simulink model "my_gm_HDLPayloadFull"  (R2024a)
settings: Solver=FixedStepDiscrete  StartTime=0.0  StopTime=stopTime  RelTol=1e-3
values from neighbouring files (symbols this model uses):
  pWords = [pWords binl2str(pBitsRaw{i})]    [testPayloadFull.m]
undefined symbols (not defined in the file or in its folder): fs, msgIn
libraries: hdlmdlgenlib x66, hdlsllib x16, dspsrcs4 x9, dspsigops x9, simulink x4, whdlutilities x4, whdledac x1
(part 1 of 2)
settings Model: SimulationMode=accelerator  Creator=cotti  LastModifiedBy=cotti
settings OptimizationCC: BlockReduction=off  ConditionallyExecuteInputs=off  DefaultParameterBehavior=Inlined  InheritOutputTypeSmallerThanSingle=on
settings DebuggingCC: AlgebraicLoopMsg=error  ArtificialAlgebraicLoopMsg=error  InheritedTsInSrcMsg=none  SingleTaskRateTransMsg=error  UnconnectedInputMsg=warning  UnconnectedOutputMsg=warning  UnconnectedLineMsg=warning
settings HardwareCC: ProdBitPerPointer=32  ProdBitPerSizeT=32  ProdBitPerPtrDiffT=32  ProdLargestAtomicFloat=None  ProdIntDivRoundTo=Undefined  ProdEndianess=Unspecified  ProdWordSize=32  ProdHWDeviceType=ASIC/FPGA->ASIC/FPGA  TargetBitPerLong=64  TargetBitPerPointer=64  TargetBitPerSizeT=64  TargetBitPerPtrDiffT=64  TargetLongLongMode=on  TargetIntDivRoundTo=Zero  TargetEndianess=LittleEndian  TargetWordSize=64  TargetHWDeviceType=Custom Processor->MATLAB Host Computer  ProdEqTarget=off

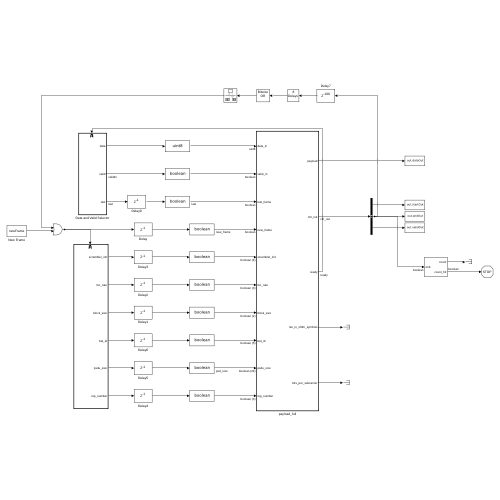
[thumbnail: Simulink's stored preview of the top-level diagram]
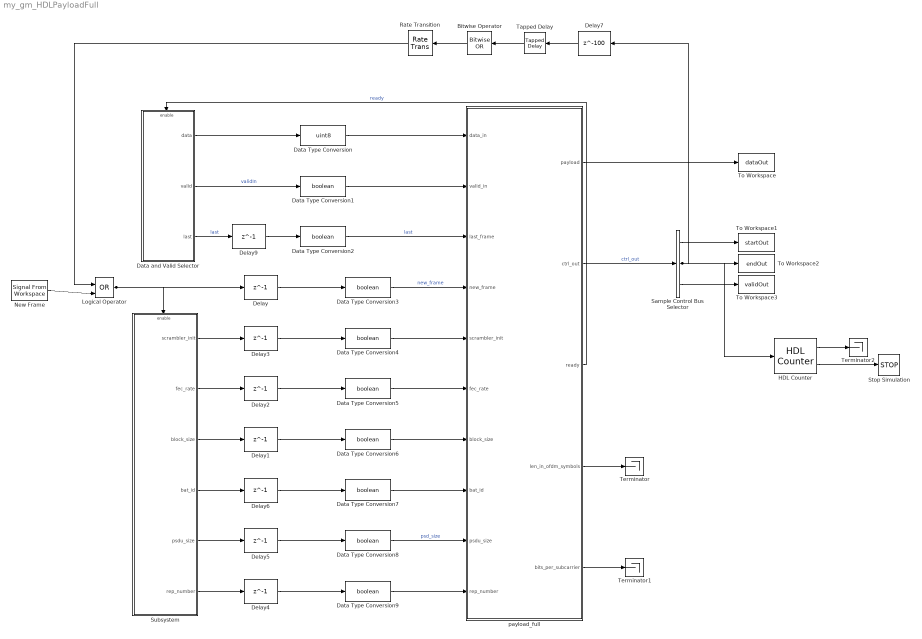
== system my_gm_HDLPayloadFull ==
  Bitwise Operator : simulink/Logic and Bit Operations/Bitwise Operator  logicop=OR  UseBitMask=off  BitMask=bin2dec('11011001')  BitMaskRealWorld=Stored Integer
      settings: LibrarySourceBlock=|
      | hdlsllib/Logic and Bit
      | Operations/Bitwise
      | Operator
  Data Type Conversion : DataTypeConversion  OutDataTypeStr=uint8  SaturateOnIntegerOverflow=off  RndMeth=Floor
  Data Type Conversion{1..9} (9 alike) : DataTypeConversion  OutDataTypeStr=boolean  SaturateOnIntegerOverflow=off  RndMeth=Floor
  Data and Valid Selector : Subsystem  TreatAsAtomicUnit=on
  Delay{,1..6,9} (8 alike) : Delay  DelayLength=1  InitialCondition=0  UseCircularBuffer=on
  Delay7 : Delay  DelayLength=100  InitialCondition=0  UseCircularBuffer=on
  HDL Counter : hdlsllib/Sources/HDL Counter  CountType=Count limited  CountInit=0  CountStep=1  CountMax=length(msgIn)  CountFromType=Initial value  CountFrom=0  CountResetPort=off  CountLoadPort=off  CountEnbPort=on  CountDirPort=off  CountHitOutputPort=on  CountDataType=Unsigned  CountWordLen=8  CountFracLen=0  CountSampTime=1
  Logical Operator : Logic  Operator=OR  IconShape=distinctive  AllPortsSameDT=off  OutDataTypeStr=boolean
  New Frame : dspsrcs4/Signal From Workspace  X=newFrame  Ts=8/fs  nsamps=1  OutputAfterFinalValue=Setting to zero  ignoreOrWarnInputAndFrameLengths=off  OutputFrames=off
  Rate Transition : RateTransition  OutPortSampleTimeOpt=Multiple of input port sample time  OutPortSampleTimeMultiple=8
  Sample Control Bus Selector : whdlutilities/Sample Control Bus Selector  OutputSignals=start,end,valid
  Stop Simulation : Stop
  Subsystem : Subsystem
  Tapped Delay : simulink/Discrete/Tapped Delay  vinit=0.0  samptime=-1  NumDelays=8  DelayOrder=Oldest  includeCurrent=off
      settings: LibrarySourceBlock=hdlsllib/Discrete/Tapped Delay
  Terminator : Terminator
  Terminator1 : Terminator
  Terminator2 : Terminator
  To Workspace : ToWorkspace  VariableName=dataOut  SampleTime=1/fs
      settings: Save2DSignal=2-D array (concatenate along first dimension)
  To Workspace1 : ToWorkspace  VariableName=startOut  SampleTime=1/fs
      settings: Save2DSignal=2-D array (concatenate along first dimension)
  To Workspace2 : ToWorkspace  VariableName=endOut  SampleTime=1/fs
      settings: Save2DSignal=2-D array (concatenate along first dimension)
  To Workspace3 : ToWorkspace  VariableName=validOut  SampleTime=1/fs
      settings: Save2DSignal=2-D array (concatenate along first dimension)
  payload_full : Subsystem  TreatAsAtomicUnit=on
  wires:
  Delay7/1 -> Tapped Delay/1
  Data Type Conversion2/1 -> payload_full/3(last_frame)  "last"
  Subsystem/6(rep_number) -> Delay4/1
  Subsystem/5(psdu_size) -> Delay5/1
  Subsystem/4(bat_id) -> Delay6/1
  Subsystem/3(block_size) -> Delay1/1
  Subsystem/2(fec_rate) -> Delay2/1
  Subsystem/1(scrambler_init) -> Delay3/1
  Tapped Delay/1 -> Bitwise Operator/1
  Rate Transition/1 -> Logical Operator/1
  Bitwise Operator/1 -> Rate Transition/1
  New Frame/1 -> Logical Operator/2
  Logical Operator/1 -> Delay/1, Subsystem/Enable
  HDL Counter/1 -> Terminator2/1
  HDL Counter/2 -> Stop Simulation/1
  Delay9/1 -> Data Type Conversion2/1
  Data and Valid Selector/1(data) -> Data Type Conversion/1
  Delay6/1 -> Data Type Conversion7/1
  Data Type Conversion9/1 -> payload_full/10(rep_number)
  Delay4/1 -> Data Type Conversion9/1
  Data and Valid Selector/2(valid) -> Data Type Conversion1/1  "validIn"
  Data Type Conversion6/1 -> payload_full/7(block_size)
  Delay/1 -> Data Type Conversion3/1
  Data Type Conversion3/1 -> payload_full/4(new_frame)  "new_frame"
  Data Type Conversion4/1 -> payload_full/5(scrambler_init)
  Data Type Conversion1/1 -> payload_full/2(valid_in)
  Data Type Conversion5/1 -> payload_full/6(fec_rate)
  Delay3/1 -> Data Type Conversion4/1
  Data and Valid Selector/3(last) -> Delay9/1  "last"
  Delay2/1 -> Data Type Conversion5/1
  payload_full/3(ready) -> Data and Valid Selector/Enable  "ready"
  payload_full/5(bits_per_subcarrier) -> Terminator1/1
  Data Type Conversion8/1 -> payload_full/9(psdu_size)  "psd_size"
  Delay5/1 -> Data Type Conversion8/1
  payload_full/1(payload) -> To Workspace/1
  Sample Control Bus Selector/2 -> To Workspace2/1, HDL Counter/1, Delay7/1
  Sample Control Bus Selector/3 -> To Workspace3/1
  Sample Control Bus Selector/1 -> To Workspace1/1
  Data Type Conversion/1 -> payload_full/1(data_in)
  Delay1/1 -> Data Type Conversion6/1
  payload_full/4(len_in_ofdm_symbols) -> Terminator/1
  Data Type Conversion7/1 -> payload_full/8(bat_id)
  payload_full/2(ctrl_out) -> Sample Control Bus Selector/1  "ctrl_out"

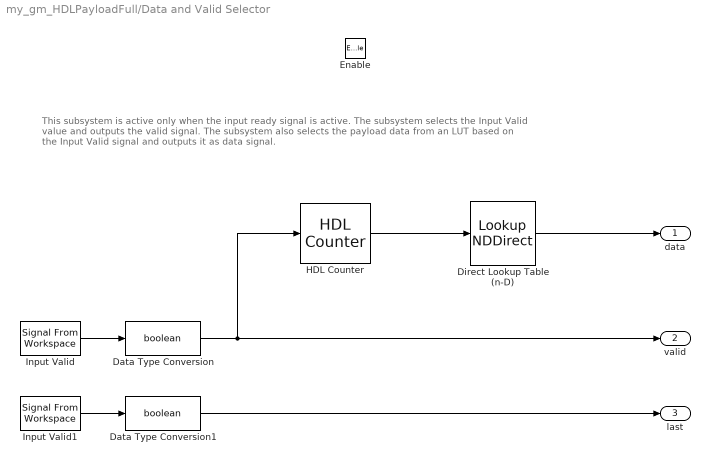
== system my_gm_HDLPayloadFull/Data and Valid Selector ==
  note: This subsystem is active only when the input ready signal is active. The subsystem selects the Input Valid value and outputs the valid signal.
      | The subsystem also selects the payload data from an LUT based on the Input Valid signal and outputs it as data signal.
  Enable : EnablePort
  Data Type Conversion : DataTypeConversion  OutDataTypeStr=boolean  SaturateOnIntegerOverflow=off  RndMeth=Floor
  Data Type Conversion1 : DataTypeConversion  OutDataTypeStr=boolean  SaturateOnIntegerOverflow=off  RndMeth=Floor
  Direct Lookup Table (n-D) : LookupNDDirect  NumberOfTableDimensions=1  Table=uint8(pWords')  DiagnosticForOutOfRangeInput=Error  TableDataTypeStr=uint8
  HDL Counter : hdlsllib/Sources/HDL Counter  CountType=Count limited  CountInit=0  CountStep=1  CountMax=length(pWords) -1  CountFromType=Initial value  CountFrom=0  CountResetPort=off  CountLoadPort=off  CountEnbPort=on  CountDirPort=off  CountHitOutputPort=off  CountDataType=Unsigned  CountWordLen=nextpow2(length(pWords))  CountFracLen=0  CountSampTime=1
  Input Valid : dspsrcs4/Signal From Workspace  X=validIn  Ts=8/fs  nsamps=1  OutputAfterFinalValue=Setting to zero  ignoreOrWarnInputAndFrameLengths=off  OutputFrames=off
  Input Valid1 : dspsrcs4/Signal From Workspace  X=lastIn  Ts=8/fs  nsamps=1  OutputAfterFinalValue=Setting to zero  ignoreOrWarnInputAndFrameLengths=off  OutputFrames=off
  data : Outport  InitialOutput=0  VectorParamsAs1DForOutWhenUnconnected=off
  valid : Outport  Port=2  InitialOutput=0  VectorParamsAs1DForOutWhenUnconnected=off
  last : Outport  Port=3  VectorParamsAs1DForOutWhenUnconnected=off
  wires:
  Data Type Conversion1/1 -> last/1
  Input Valid1/1 -> Data Type Conversion1/1
  Data Type Conversion/1 -> HDL Counter/1, valid/1
  Input Valid/1 -> Data Type Conversion/1
  Direct Lookup Table (n-D)/1 -> data/1
  HDL Counter/1 -> Direct Lookup Table (n-D)/1

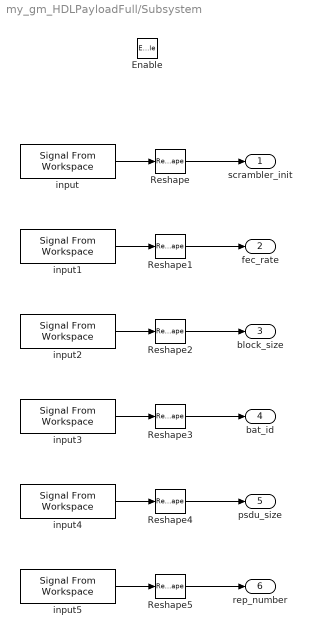
== system my_gm_HDLPayloadFull/Subsystem ==
  Enable : EnablePort
  Reshape{,1..5} (6 alike) : Reshape
  input : dspsrcs4/Signal From Workspace  X=scramblerInitLSB  Ts=8/fs  nsamps=1  OutputAfterFinalValue=Setting to zero  ignoreOrWarnInputAndFrameLengths=off  OutputFrames=off
  input1 : dspsrcs4/Signal From Workspace  X=fecRateLSB  Ts=8/fs  nsamps=1  OutputAfterFinalValue=Setting to zero  ignoreOrWarnInputAndFrameLengths=off  OutputFrames=off
  input2 : dspsrcs4/Signal From Workspace  X=blockSizeLSB  Ts=8/fs  nsamps=1  OutputAfterFinalValue=Setting to zero  ignoreOrWarnInputAndFrameLengths=off  OutputFrames=off
  input3 : dspsrcs4/Signal From Workspace  X=batIdLSB  Ts=8/fs  nsamps=1  OutputAfterFinalValue=Setting to zero  ignoreOrWarnInputAndFrameLengths=off  OutputFrames=off
  input4 : dspsrcs4/Signal From Workspace  X=psduSizeLSB  Ts=8/fs  nsamps=1  OutputAfterFinalValue=Setting to zero  ignoreOrWarnInputAndFrameLengths=off  OutputFrames=off
  input5 : dspsrcs4/Signal From Workspace  X=repNumberLSB  Ts=8/fs  nsamps=1  OutputAfterFinalValue=Setting to zero  ignoreOrWarnInputAndFrameLengths=off  OutputFrames=off
  scrambler_init : Outport
  fec_rate : Outport  Port=2
  block_size : Outport  Port=3
  bat_id : Outport  Port=4
  psdu_size : Outport  Port=5
  rep_number : Outport  Port=6
  wires:
  Reshape5/1 -> rep_number/1
  Reshape4/1 -> psdu_size/1
  Reshape3/1 -> bat_id/1
  Reshape2/1 -> block_size/1
  Reshape1/1 -> fec_rate/1
  Reshape/1 -> scrambler_init/1
  input4/1 -> Reshape4/1
  input1/1 -> Reshape1/1
  input2/1 -> Reshape2/1
  input5/1 -> Reshape5/1
  input3/1 -> Reshape3/1
  input/1 -> Reshape/1

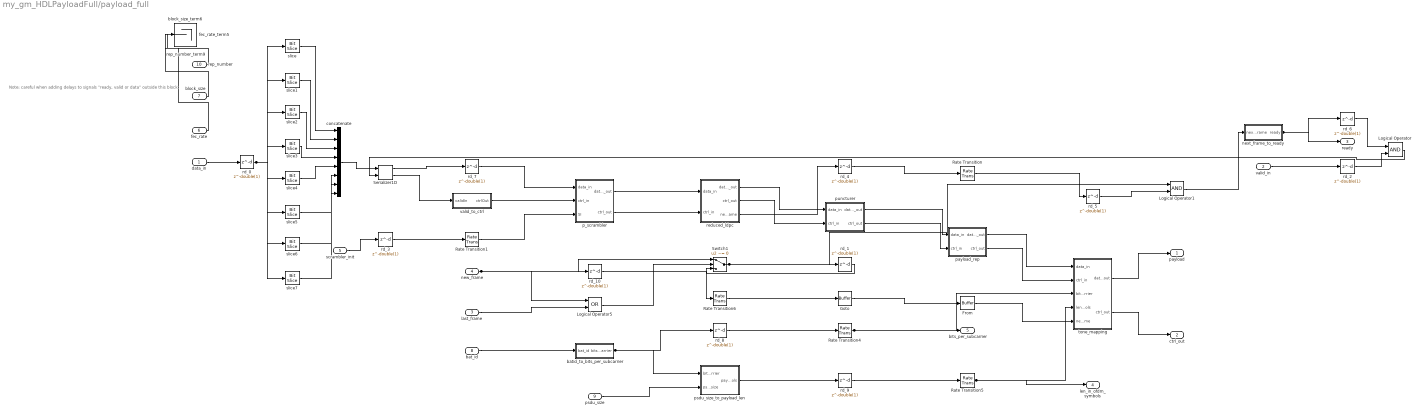
== system my_gm_HDLPayloadFull/payload_full ==
  note: Note: careful when adding delays to signals "ready, valid or data" outside this block
  data_in : Inport  OutDataTypeStr=uint8  PortDimensions=1  SampleTime=8e-08
  valid_in : Inport  Port=2  OutDataTypeStr=boolean  PortDimensions=1  SampleTime=8e-08
  last_frame : Inport  Port=3  OutDataTypeStr=boolean  PortDimensions=1  SampleTime=8e-08
  new_frame : Inport  Port=4  OutDataTypeStr=boolean  PortDimensions=1  SampleTime=8e-08
  scrambler_init : Inport  Port=5  OutDataTypeStr=boolean  PortDimensions=[4]  SampleTime=8e-08
  fec_rate : Inport  Port=6  OutDataTypeStr=boolean  PortDimensions=[3]  SampleTime=8e-08
  block_size : Inport  Port=7  OutDataTypeStr=boolean  PortDimensions=[2]  SampleTime=8e-08
  bat_id : Inport  Port=8  OutDataTypeStr=boolean  PortDimensions=[5]  SampleTime=8e-08
  psdu_size : Inport  Port=9  OutDataTypeStr=boolean  PortDimensions=[24]  SampleTime=8e-08
  rep_number : Inport  Port=10  OutDataTypeStr=boolean  PortDimensions=[3]  SampleTime=8e-08
  From : hdlmdlgenlib/Buffer
  Goto : hdlmdlgenlib/Buffer
  Logical Operator : Logic  AllPortsSameDT=off  OutDataTypeStr=boolean  SampleTime=8e-08
  Logical Operator1 : Logic  AllPortsSameDT=off  OutDataTypeStr=boolean  SampleTime=8e-08
  Logical Operator5 : Logic  Operator=OR  AllPortsSameDT=off  OutDataTypeStr=boolean  SampleTime=8e-08
  Rate Transition : RateTransition  InitialCondition=double(0)  OutPortSampleTimeOpt=Multiple of input port sample time  OutPortSampleTimeMultiple=8
  Rate Transition1 : RateTransition  Integrity=off  Deterministic=off  OutPortSampleTimeOpt=Multiple of input port sample time  OutPortSampleTimeMultiple=1/8
  Rate Transition4 : RateTransition  Integrity=off  Deterministic=off  InitialCondition="fi(0,0,4,0,\"hex\",\"0\")"  OutPortSampleTimeOpt=Multiple of input port sample time  OutPortSampleTimeMultiple=1/8
  Rate Transition5 : RateTransition  Integrity=off  Deterministic=off  OutPortSampleTimeOpt=Multiple of input port sample time  OutPortSampleTimeMultiple=1/8
  Rate Transition6 : RateTransition  Integrity=off  Deterministic=off  OutPortSampleTimeOpt=Multiple of input port sample time  OutPortSampleTimeMultiple=1/8
  Serializer1D : hdlsllib/HDL Operations/Serializer1D  Ratio=8  IdleCycles=0  validIn=on  startOut=off  validOut=on  inputDataDimensions=8  inputSampleTime=8e-08  inputSignalType=real
  Switch1 : Switch  Criteria=u2 ~= 0  Threshold=double(0)  OutDataTypeStr=boolean  SampleTime=8e-08  SaturateOnIntegerOverflow=off  InputSameDT=off
  batid_to_bits_per_subcarrier : Subsystem
  block_size_term6 : Terminator
  concatenate : Concatenate  NumInputs=8  Mode=Multidimensional array  ConcatenateDimension=2
  fec_rate_term5 : Terminator
  next_frame_to_ready : Subsystem
  p_scrambler : Subsystem
  payload_rep : Subsystem
  psdu_size_to_payload_len : Subsystem
  puncturer : Subsystem
  rd_{0..3,5..6,8..10} (9 alike) : Delay  DelayLength=double(1)  InitialCondition=0  SampleTime=8e-08
  rd_4 : Delay  DelayLength=double(1)  InitialCondition=0  SampleTime=1e-08
  rd_7 : Delay  DelayLength=double(1)  InitialCondition=0  SampleTime=1e-08
  reduced_ldpc : Subsystem
  rep_number_term9 : Terminator
  slice : hdlsllib/Logic and Bit Operations/Bit Slice  lidx=double(0)  ridx=double(0)
  slice1 : hdlsllib/Logic and Bit Operations/Bit Slice  lidx=double(1)  ridx=double(1)
  slice2 : hdlsllib/Logic and Bit Operations/Bit Slice  lidx=double(2)  ridx=double(2)
  slice3 : hdlsllib/Logic and Bit Operations/Bit Slice  lidx=double(3)  ridx=double(3)
  slice4 : hdlsllib/Logic and Bit Operations/Bit Slice  lidx=double(4)  ridx=double(4)
  slice5 : hdlsllib/Logic and Bit Operations/Bit Slice  lidx=double(5)  ridx=double(5)
  slice6 : hdlsllib/Logic and Bit Operations/Bit Slice  lidx=double(6)  ridx=double(6)
  slice7 : hdlsllib/Logic and Bit Operations/Bit Slice  lidx=double(7)  ridx=double(7)
  tone_mapping : Subsystem
  valid_to_ctrl : Subsystem
  payload : Outport  SampleTime=1e-08  VectorParamsAs1DForOutWhenUnconnected=off
  ctrl_out : Outport  Port=2  VectorParamsAs1DForOutWhenUnconnected=off
  ready : Outport  Port=3  SampleTime=8e-08  VectorParamsAs1DForOutWhenUnconnected=off
  len_in_ofdm_symbols : Outport  Port=4  SampleTime=1e-08  VectorParamsAs1DForOutWhenUnconnected=off
  bits_per_subcarrier : Outport  Port=5  SampleTime=1e-08  VectorParamsAs1DForOutWhenUnconnected=off
  wires:
  valid_in/1 -> rd_2/1
  last_frame/1 -> Logical Operator5/2
  new_frame/1 -> rd_10/1, Logical Operator5/1, Switch1/1
  scrambler_init/1 -> rd_3/1
  fec_rate/1 -> fec_rate_term5/1
  block_size/1 -> block_size_term6/1
  bat_id/1 -> batid_to_bits_per_subcarrier/1(bat_id)
  psdu_size/1 -> psdu_size_to_payload_len/2(psdu_size)
  rep_number/1 -> rep_number_term9/1
  From/1 -> tone_mapping/5(new_frame)
  Rate Transition4/1 -> tone_mapping/3(bits_per_subcarrier), bits_per_subcarrier/1
  Rate Transition5/1 -> tone_mapping/4(len_in_ofdm_symbols), len_in_ofdm_symbols/1
  batid_to_bits_per_subcarrier/1(bits_per_subcarrier) -> rd_8/1, psdu_size_to_payload_len/1(bits_per_subcarrier)
  next_frame_to_ready/1(ready) -> rd_6/1, ready/1
  payload_rep/1(data_out) -> tone_mapping/1(data_in)
  payload_rep/2(ctrl_out) -> tone_mapping/2(ctrl_in)
  psdu_size_to_payload_len/1(payload_len_in_ofdm_symbols) -> rd_9/1
  reduced_ldpc/1(data_out) -> puncturer/1(data_in)
  reduced_ldpc/2(ctrl_out) -> puncturer/2(ctrl_in)
  tone_mapping/1(data_out) -> payload/1
  tone_mapping/2(ctrl_out) -> ctrl_out/1
  Rate Transition6/1 -> Goto/1
  Switch1/1 -> rd_1/1, Logical Operator1/1
  puncturer/1(data_out) -> payload_rep/1(data_in)
  puncturer/2(ctrl_out) -> payload_rep/2(ctrl_in)
  Goto/1 -> From/1
  concatenate/1 -> Serializer1D/1
  slice/1 -> concatenate/1
  slice1/1 -> concatenate/2
  slice2/1 -> concatenate/3
  slice3/1 -> concatenate/4
  slice4/1 -> concatenate/5
  slice5/1 -> concatenate/6
  slice6/1 -> concatenate/7
  slice7/1 -> concatenate/8
  Logical Operator5/1 -> Switch1/2
  p_scrambler/1(data_out) -> reduced_ldpc/1(data_in)
  valid_to_ctrl/1(ctrlOut) -> p_scrambler/2(ctrl_in)
  p_scrambler/2(ctrl_out) -> reduced_ldpc/2(ctrl_in)
  Rate Transition1/1 -> p_scrambler/3(SI)
  Serializer1D/1 -> rd_7/1
  Serializer1D/2 -> valid_to_ctrl/1(validIn)
  Logical Operator/1 -> Serializer1D/2
  reduced_ldpc/3(next_frame) -> rd_4/1
  Rate Transition/1 -> rd_5/1
  Logical Operator1/1 -> next_frame_to_ready/1(next_frame)
  rd_8/1 -> Rate Transition4/1
  rd_9/1 -> Rate Transition5/1
  rd_10/1 -> Rate Transition6/1
  rd_2/1 -> Logical Operator/2
  rd_3/1 -> Rate Transition1/1
  rd_1/1 -> Switch1/3
  rd_7/1 -> p_scrambler/1(data_in)
  rd_4/1 -> Rate Transition/1
  rd_5/1 -> Logical Operator1/2
  rd_6/1 -> Logical Operator/1
  data_in/1 -> rd_0/1
  rd_0/1 -> slice/1, slice1/1, slice2/1, slice3/1, slice4/1, slice5/1, slice6/1, slice7/1

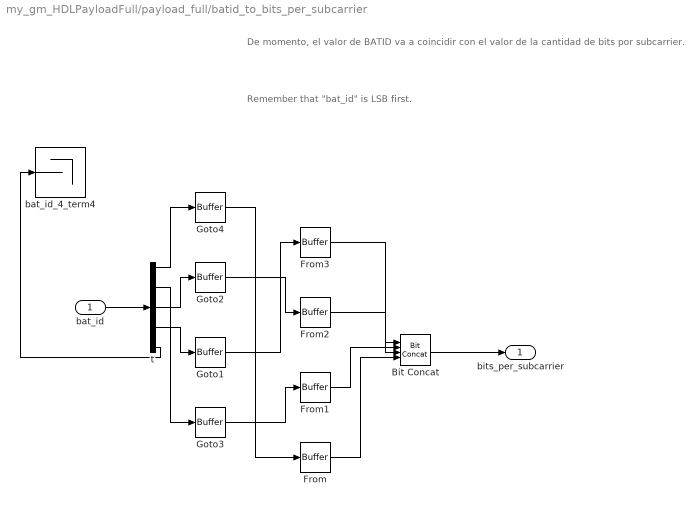
== system my_gm_HDLPayloadFull/payload_full/batid_to_bits_per_subcarrier ==
  note: De momento, el valor de BATID va a coincidir con el valor de la cantidad de bits por subcarrier.
  note: Remember that "bat_id" is LSB first.
  bat_id : Inport  OutDataTypeStr=boolean  PortDimensions=[5]  SampleTime=8e-08
  Bit Concat : hdlsllib/Logic and Bit Operations/Bit Concat  numInputs=4
  From{,1..3} (4 alike) : hdlmdlgenlib/Buffer
  Goto{1..4} (4 alike) : hdlmdlgenlib/Buffer
  bat_id_4_term4 : Terminator
  t : Demux  Outputs=5
  bits_per_subcarrier : Outport  SampleTime=8e-08
  wires:
  bat_id/1 -> t/1
  Bit Concat/1 -> bits_per_subcarrier/1
  From/1 -> Bit Concat/4
  From1/1 -> Bit Concat/3
  From2/1 -> Bit Concat/2
  From3/1 -> Bit Concat/1
  Goto4/1 -> From/1
  Goto3/1 -> From1/1
  Goto2/1 -> From2/1
  Goto1/1 -> From3/1
  t/1 -> Goto4/1
  t/2 -> Goto3/1
  t/3 -> Goto2/1
  t/4 -> Goto1/1
  t/5 -> bat_id_4_term4/1

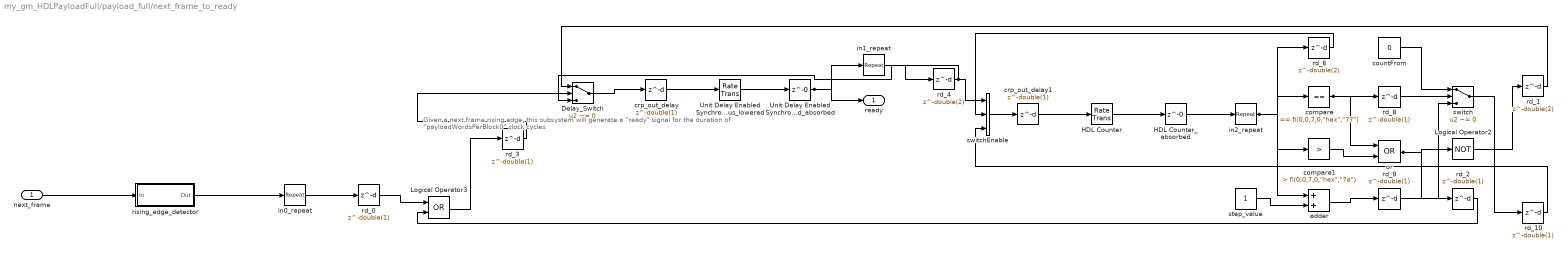
== system my_gm_HDLPayloadFull/payload_full/next_frame_to_ready ==
  note: Given a next frame rising edge, this subsystem will generate a "ready" signal for the duration of "payloadWordsPerBlock0" clock cycles
  next_frame : Inport  OutDataTypeStr=boolean  SampleTime=8e-08
  Delay_Switch : Switch  Criteria=u2 ~= 0  Threshold=double(0)  OutDataTypeStr=boolean  SampleTime=1e-08  SaturateOnIntegerOverflow=off  InputSameDT=off
  HDL Counter : RateTransition  OutPortSampleTimeOpt=Multiple of input port sample time  OutPortSampleTimeMultiple=8
  HDL Counter_absorbed : Delay  DelayLength=0
  Logical Operator2 : Logic  Operator=NOT  Inputs=1  AllPortsSameDT=off  OutDataTypeStr=boolean  SampleTime=1e-08
  Logical Operator3 : Logic  Operator=OR  AllPortsSameDT=off  OutDataTypeStr=boolean  SampleTime=1e-08
  Unit Delay Enabled Synchronous_lowered : RateTransition  OutPortSampleTimeOpt=Multiple of input port sample time  OutPortSampleTimeMultiple=8
  Unit Delay Enabled Synchronous_lowered_absorbed : Delay  DelayLength=0
  adder : Sum  OutDataTypeStr=fixdt(0, 7, 0)  AccumDataTypeStr=fixdt(0, 7, 0)  SampleTime=1e-08
  compare : simulink/Logic and Bit Operations/Compare To Constant  relop===  const="fi(0,0,7,0,\"hex\",\"77\")"  OutDataTypeStr=boolean
  compare1 : simulink/Logic and Bit Operations/Compare To Constant  relop=>  const="fi(0,0,7,0,\"hex\",\"7e\")"  OutDataTypeStr=boolean
  countFrom : Constant  Value=0  VectorParams1D=off  OutDataTypeStr=fixdt(0, 7, 0)  SampleTime=1e-08
  crp_out_delay : Delay  DelayLength=double(1)  InitialCondition=0  SampleTime=1e-08
  crp_out_delay1 : Delay  DelayLength=double(1)  InitialCondition=0  SampleTime=1e-08
  in0_repeat : dspsigops/Repeat  FactorSource=Dialog parameter  N=double(8)  Nmax=16  RateOptions=Allow multirate processing  ic=0  mode=Unused parameter value
  in1_repeat : dspsigops/Repeat  FactorSource=Dialog parameter  N=double(8)  Nmax=16  RateOptions=Allow multirate processing  ic=0  mode=Unused parameter value
  in2_repeat : dspsigops/Repeat  FactorSource=Dialog parameter  N=double(8)  Nmax=16  RateOptions=Allow multirate processing  ic=0  mode=Unused parameter value
  or : Logic  Operator=OR  AllPortsSameDT=off  OutDataTypeStr=boolean  SampleTime=1e-08
  rd_{0,2..3,8..10} (6 alike) : Delay  DelayLength=double(1)  InitialCondition=0  SampleTime=1e-08
  rd_1 : Delay  DelayLength=double(2)  InitialCondition=0  SampleTime=1e-08
  rd_4 : Delay  DelayLength=double(2)  InitialCondition=0  SampleTime=1e-08
  rd_6 : Delay  DelayLength=double(2)  InitialCondition=0  SampleTime=1e-08
  rising_edge_detector : Subsystem
  step_value : Constant  VectorParams1D=off  OutDataTypeStr=fixdt(0, 7, 0)  SampleTime=1e-08
  switch : Switch  Criteria=u2 ~= 0  Threshold=double(0)  OutDataTypeStr=fixdt(0, 7, 0)  SampleTime=1e-08  SaturateOnIntegerOverflow=off  InputSameDT=off
  switchEnable : MultiPortSwitch  DataPortOrder=Zero-based contiguous  Inputs=2  DiagnosticForDefault=None  zeroidx=on  OutDataTypeStr=fixdt(0, 7, 0)  SampleTime=1e-08  SaturateOnIntegerOverflow=off  InputSameDT=off
  ready : Outport  SampleTime=8e-08
  wires:
  next_frame/1 -> rising_edge_detector/1(In)
  rising_edge_detector/1(Out) -> in0_repeat/1
  Unit Delay Enabled Synchronous_lowered_absorbed/1 -> ready/1, in1_repeat/1
  in0_repeat/1 -> rd_0/1
  HDL Counter/1 -> HDL Counter_absorbed/1
  HDL Counter_absorbed/1 -> in2_repeat/1
  in2_repeat/1 -> rd_6/1, adder/1, compare/1, compare1/1
  in1_repeat/1 -> rd_4/1
  crp_out_delay/1 -> Unit Delay Enabled Synchronous_lowered/1
  crp_out_delay1/1 -> HDL Counter/1
  Unit Delay Enabled Synchronous_lowered/1 -> Unit Delay Enabled Synchronous_lowered_absorbed/1
  switchEnable/1 -> crp_out_delay1/1
  countFrom/1 -> switch/1
  step_value/1 -> adder/2
  adder/1 -> rd_9/1
  switch/1 -> rd_10/1
  compare/1 -> rd_8/1, or/1
  compare1/1 -> or/2
  or/1 -> rd_2/1, Logical Operator2/1
  Logical Operator3/1 -> rd_3/1
  Delay_Switch/1 -> crp_out_delay/1
  Logical Operator2/1 -> rd_1/1
  rd_6/1 -> switchEnable/2
  rd_1/1 -> Delay_Switch/1
  rd_0/1 -> Logical Operator3/1
  rd_2/1 -> Logical Operator3/2
  rd_3/1 -> Delay_Switch/2
  rd_9/1 -> switch/3
  rd_10/1 -> switchEnable/3
  rd_8/1 -> switch/2
  rd_4/1 -> Delay_Switch/3, switchEnable/1

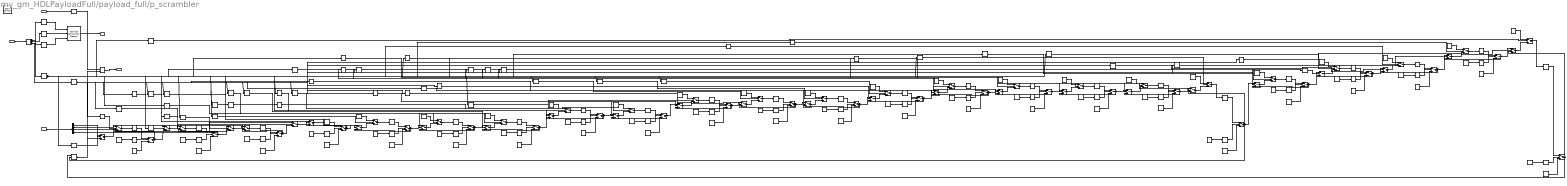
== system my_gm_HDLPayloadFull/payload_full/p_scrambler ==
  data_in : Inport  OutDataTypeStr=fixdt(0, 1, 0)  SampleTime=1e-08
  ctrl_in : Inport  Port=2  SampleTime=1e-08
  SI : Inport  Port=3  OutDataTypeStr=boolean  PortDimensions=[4]  SampleTime=1e-08
  C10_lowered : Delay  DelayLength=double(1)  InitialCondition=0  SampleTime=1e-08
  C10_lowered_Initial_Val : Constant  Value=double(1)  OutDataTypeStr=boolean  SampleTime=1e-08
  C10_lowered_ctrl_const : Constant  OutDataTypeStr=boolean  SampleTime=1e-08
  C10_lowered_ctrl_delay : Delay  DelayLength=double(1)  InitialCondition=0  SampleTime=1e-08
  C10_lowered_switch : Switch  Criteria=u2 ~= 0  Threshold=double(0)  OutDataTypeStr=boolean  SampleTime=1e-08  SaturateOnIntegerOverflow=off  InputSameDT=off
  C11_lowered : Delay  DelayLength=double(1)  InitialCondition=0  SampleTime=1e-08
  C11_lowered_Initial_Val : Constant  Value=double(1)  OutDataTypeStr=boolean  SampleTime=1e-08
  C11_lowered_ctrl_const : Constant  OutDataTypeStr=boolean  SampleTime=1e-08
  C11_lowered_ctrl_delay : Delay  DelayLength=double(1)  InitialCondition=0  SampleTime=1e-08
  C11_lowered_switch : Switch  Criteria=u2 ~= 0  Threshold=double(0)  OutDataTypeStr=boolean  SampleTime=1e-08  SaturateOnIntegerOverflow=off  InputSameDT=off
  C12_lowered : Delay  DelayLength=double(1)  InitialCondition=0  SampleTime=1e-08
  C12_lowered_Initial_Val : Constant  Value=double(1)  OutDataTypeStr=boolean  SampleTime=1e-08
  C12_lowered_ctrl_const : Constant  OutDataTypeStr=boolean  SampleTime=1e-08
  C12_lowered_ctrl_delay : Delay  DelayLength=double(1)  InitialCondition=0  SampleTime=1e-08
  C12_lowered_switch : Switch  Criteria=u2 ~= 0  Threshold=double(0)  OutDataTypeStr=boolean  SampleTime=1e-08  SaturateOnIntegerOverflow=off  InputSameDT=off
  C13_lowered : Delay  DelayLength=double(1)  InitialCondition=0  SampleTime=1e-08
  C13_lowered_Initial_Val : Constant  Value=double(1)  OutDataTypeStr=boolean  SampleTime=1e-08
  C13_lowered_ctrl_const : Constant  OutDataTypeStr=boolean  SampleTime=1e-08
  C13_lowered_ctrl_delay : Delay  DelayLength=double(1)  InitialCondition=0  SampleTime=1e-08
  C13_lowered_switch : Switch  Criteria=u2 ~= 0  Threshold=double(0)  OutDataTypeStr=boolean  SampleTime=1e-08  SaturateOnIntegerOverflow=off  InputSameDT=off
  C14_lowered : Delay  DelayLength=double(1)  InitialCondition=0  SampleTime=1e-08
  C14_lowered_Initial_Val : Constant  Value=double(1)  OutDataTypeStr=boolean  SampleTime=1e-08
  C14_lowered_ctrl_const : Constant  OutDataTypeStr=boolean  SampleTime=1e-08
  C14_lowered_ctrl_delay : Delay  DelayLength=double(1)  InitialCondition=0  SampleTime=1e-08
  C14_lowered_switch : Switch  Criteria=u2 ~= 0  Threshold=double(0)  OutDataTypeStr=boolean  SampleTime=1e-08  SaturateOnIntegerOverflow=off  InputSameDT=off
  C15_lowered : Delay  DelayLength=double(1)  InitialCondition=0  SampleTime=1e-08
  C15_lowered_Initial_Val : Constant  Value=double(1)  OutDataTypeStr=boolean  SampleTime=1e-08
  C15_lowered_ctrl_const : Constant  OutDataTypeStr=boolean  SampleTime=1e-08
  C15_lowered_ctrl_delay : Delay  DelayLength=double(1)  InitialCondition=0  SampleTime=1e-08
  C15_lowered_switch : Switch  Criteria=u2 ~= 0  Threshold=double(0)  OutDataTypeStr=boolean  SampleTime=1e-08  SaturateOnIntegerOverflow=off  InputSameDT=off
  C16_lowered : Delay  DelayLength=double(1)  InitialCondition=0  SampleTime=1e-08
  C16_lowered_Initial_Val : Constant  Value=double(1)  OutDataTypeStr=boolean  SampleTime=1e-08
  C16_lowered_ctrl_const : Constant  OutDataTypeStr=boolean  SampleTime=1e-08
  C16_lowered_ctrl_delay : Delay  DelayLength=double(1)  InitialCondition=0  SampleTime=1e-08
  C16_lowered_switch : Switch  Criteria=u2 ~= 0  Threshold=double(0)  OutDataTypeStr=boolean  SampleTime=1e-08  SaturateOnIntegerOverflow=off  InputSameDT=off
  C17_lowered : Delay  DelayLength=double(1)  InitialCondition=0  SampleTime=1e-08
  C17_lowered_Initial_Val : Constant  Value=double(1)  OutDataTypeStr=boolean  SampleTime=1e-08
  C17_lowered_ctrl_const : Constant  OutDataTypeStr=boolean  SampleTime=1e-08
  C17_lowered_ctrl_delay : Delay  DelayLength=double(1)  InitialCondition=0  SampleTime=1e-08
  C17_lowered_switch : Switch  Criteria=u2 ~= 0  Threshold=double(0)  OutDataTypeStr=boolean  SampleTime=1e-08  SaturateOnIntegerOverflow=off  InputSameDT=off
  C18_lowered : Delay  DelayLength=double(1)  InitialCondition=0  SampleTime=1e-08
  C18_lowered_Initial_Val : Constant  Value=double(1)  OutDataTypeStr=boolean  SampleTime=1e-08
  C18_lowered_ctrl_const : Constant  OutDataTypeStr=boolean  SampleTime=1e-08
  C18_lowered_ctrl_delay : Delay  DelayLength=double(1)  InitialCondition=0  SampleTime=1e-08
  C18_lowered_switch : Switch  Criteria=u2 ~= 0  Threshold=double(0)  OutDataTypeStr=boolean  SampleTime=1e-08  SaturateOnIntegerOverflow=off  InputSameDT=off
  C19_lowered : Delay  DelayLength=double(1)  InitialCondition=0  SampleTime=1e-08
  C19_lowered_Initial_Val : Constant  Value=double(1)  OutDataTypeStr=boolean  SampleTime=1e-08
  C19_lowered_ctrl_const : Constant  OutDataTypeStr=boolean  SampleTime=1e-08
  C19_lowered_ctrl_delay : Delay  DelayLength=double(1)  InitialCondition=0  SampleTime=1e-08
  C19_lowered_switch : Switch  Criteria=u2 ~= 0  Threshold=double(0)  OutDataTypeStr=boolean  SampleTime=1e-08  SaturateOnIntegerOverflow=off  InputSameDT=off
  C20_lowered : Delay  DelayLength=double(1)  InitialCondition=0  SampleTime=1e-08
  C20_lowered_Initial_Val : Constant  Value=double(1)  OutDataTypeStr=boolean  SampleTime=1e-08
  C20_lowered_ctrl_const : Constant  OutDataTypeStr=boolean  SampleTime=1e-08
  C20_lowered_ctrl_delay : Delay  DelayLength=double(1)  InitialCondition=0  SampleTime=1e-08
  C20_lowered_switch : Switch  Criteria=u2 ~= 0  Threshold=double(0)  OutDataTypeStr=boolean  SampleTime=1e-08  SaturateOnIntegerOverflow=off  InputSameDT=off
  C21_lowered : Delay  DelayLength=double(1)  InitialCondition=0  SampleTime=1e-08
  C21_lowered_Initial_Val : Constant  Value=double(1)  OutDataTypeStr=boolean  SampleTime=1e-08
  C21_lowered_ctrl_const : Constant  OutDataTypeStr=boolean  SampleTime=1e-08
  C21_lowered_ctrl_delay : Delay  DelayLength=double(1)  InitialCondition=0  SampleTime=1e-08
  C21_lowered_switch : Switch  Criteria=u2 ~= 0  Threshold=double(0)  OutDataTypeStr=boolean  SampleTime=1e-08  SaturateOnIntegerOverflow=off  InputSameDT=off
  C22_lowered : Delay  DelayLength=double(1)  InitialCondition=0  SampleTime=1e-08
  C22_lowered_Initial_Val : Constant  Value=double(1)  OutDataTypeStr=boolean  SampleTime=1e-08
  C22_lowered_ctrl_const : Constant  OutDataTypeStr=boolean  SampleTime=1e-08
  C22_lowered_ctrl_delay : Delay  DelayLength=double(1)  InitialCondition=0  SampleTime=1e-08
  C22_lowered_switch : Switch  Criteria=u2 ~= 0  Threshold=double(0)  OutDataTypeStr=boolean  SampleTime=1e-08  SaturateOnIntegerOverflow=off  InputSameDT=off
  C23_lowered : Delay  DelayLength=double(1)  InitialCondition=0  SampleTime=1e-08
  C23_lowered_Initial_Val : Constant  Value=double(1)  OutDataTypeStr=boolean  SampleTime=1e-08
  C23_lowered_ctrl_const : Constant  OutDataTypeStr=boolean  SampleTime=1e-08
  C23_lowered_ctrl_delay : Delay  DelayLength=double(1)  InitialCondition=0  SampleTime=1e-08
  C23_lowered_switch : Switch  Criteria=u2 ~= 0  Threshold=double(0)  OutDataTypeStr=boolean  SampleTime=1e-08  SaturateOnIntegerOverflow=off  InputSameDT=off
  C5_lowered : Delay  DelayLength=double(1)  InitialCondition=0  SampleTime=1e-08
  C5_lowered_Initial_Val : Constant  Value=double(1)  OutDataTypeStr=boolean  SampleTime=1e-08
  C5_lowered_ctrl_const : Constant  OutDataTypeStr=boolean  SampleTime=1e-08
  C5_lowered_ctrl_delay : Delay  DelayLength=double(1)  InitialCondition=0  SampleTime=1e-08
  C5_lowered_switch : Switch  Criteria=u2 ~= 0  Threshold=double(0)  OutDataTypeStr=boolean  SampleTime=1e-08  SaturateOnIntegerOverflow=off  InputSameDT=off
  C6_lowered : Delay  DelayLength=double(1)  InitialCondition=0  SampleTime=1e-08
  C6_lowered_Initial_Val : Constant  Value=double(1)  OutDataTypeStr=boolean  SampleTime=1e-08
  C6_lowered_ctrl_const : Constant  OutDataTypeStr=boolean  SampleTime=1e-08
  C6_lowered_ctrl_delay : Delay  DelayLength=double(1)  InitialCondition=0  SampleTime=1e-08
  C6_lowered_switch : Switch  Criteria=u2 ~= 0  Threshold=double(0)  OutDataTypeStr=boolean  SampleTime=1e-08  SaturateOnIntegerOverflow=off  InputSameDT=off
  C7_lowered : Delay  DelayLength=double(1)  InitialCondition=0  SampleTime=1e-08
  C7_lowered_Initial_Val : Constant  Value=double(1)  OutDataTypeStr=boolean  SampleTime=1e-08
  C7_lowered_ctrl_const : Constant  OutDataTypeStr=boolean  SampleTime=1e-08
  C7_lowered_ctrl_delay : Delay  DelayLength=double(1)  InitialCondition=0  SampleTime=1e-08
  C7_lowered_switch : Switch  Criteria=u2 ~= 0  Threshold=double(0)  OutDataTypeStr=boolean  SampleTime=1e-08  SaturateOnIntegerOverflow=off  InputSameDT=off
  C8_lowered : Delay  DelayLength=double(1)  InitialCondition=0  SampleTime=1e-08
  C8_lowered_Initial_Val : Constant  Value=double(1)  OutDataTypeStr=boolean  SampleTime=1e-08
  C8_lowered_ctrl_const : Constant  OutDataTypeStr=boolean  SampleTime=1e-08
  C8_lowered_ctrl_delay : Delay  DelayLength=double(1)  InitialCondition=0  SampleTime=1e-08
  C8_lowered_switch : Switch  Criteria=u2 ~= 0  Threshold=double(0)  OutDataTypeStr=boolean  SampleTime=1e-08  SaturateOnIntegerOverflow=off  InputSameDT=off
  C9_lowered : Delay  DelayLength=double(1)  InitialCondition=0  SampleTime=1e-08
  C9_lowered_Initial_Val : Constant  Value=double(1)  OutDataTypeStr=boolean  SampleTime=1e-08
  C9_lowered_ctrl_const : Constant  OutDataTypeStr=boolean  SampleTime=1e-08
  C9_lowered_ctrl_delay : Delay  DelayLength=double(1)  InitialCondition=0  SampleTime=1e-08
  C9_lowered_switch : Switch  Criteria=u2 ~= 0  Threshold=double(0)  OutDataTypeStr=boolean  SampleTime=1e-08  SaturateOnIntegerOverflow=off  InputSameDT=off
  Delay{1,3..5} (4 alike) : Delay  DelayLength=double(1)  InitialCondition=0  SampleTime=1e-08
  Delay_Switch{,1..3} (4 alike) : Switch  Criteria=u2 ~= 0  Threshold=double(0)  OutDataTypeStr=boolean  SampleTime=1e-08  SaturateOnIntegerOverflow=off  InputSameDT=off
  From{,1..45} (46 alike) : hdlmdlgenlib/Buffer
  Goto2 : hdlmdlgenlib/Buffer
  Goto3 : hdlmdlgenlib/Buffer
  Initial_Val{,1..18} (19 alike) : Constant  Value=double(1)  OutDataTypeStr=boolean  SampleTime=1e-08
  Logical Operator : Logic  Operator=XOR  AllPortsSameDT=off  OutDataTypeStr=boolean  SampleTime=1e-08
  Logical Operator1 : Logic  Operator=XOR  AllPortsSameDT=off  OutDataTypeStr=boolean  SampleTime=1e-08
  Sample Control Bus Creator : whdlutilities/Sample Control Bus Creator
  StateControl : StateControl  StateControl=Synchronous
  Switch{,1..3} (4 alike) : Switch  Criteria=u2 ~= 0  Threshold=double(0)  OutDataTypeStr=boolean  SampleTime=1e-08  SaturateOnIntegerOverflow=off  InputSameDT=off
  Unit Delay Enabled Synchronous1_lowered : Delay  DelayLength=double(1)  InitialCondition=0  SampleTime=1e-08
  Unit Delay Enabled Synchronous1_lowered_Initial_Val : Constant  Value=double(1)  OutDataTypeStr=boolean  SampleTime=1e-08
  Unit Delay Enabled Synchronous1_lowered_ctrl_const : Constant  OutDataTypeStr=boolean  SampleTime=1e-08
  Unit Delay Enabled Synchronous1_lowered_ctrl_delay : Delay  DelayLength=double(1)  InitialCondition=0  SampleTime=1e-08
  Unit Delay Enabled Synchronous1_lowered_switch : Switch  Criteria=u2 ~= 0  Threshold=double(0)  OutDataTypeStr=boolean  SampleTime=1e-08  SaturateOnIntegerOverflow=off  InputSameDT=off
  Unit Delay Enabled Synchronous2_lowered : Delay  DelayLength=double(1)  InitialCondition=0  SampleTime=1e-08
  Unit Delay Enabled Synchronous2_lowered_Initial_Val : Constant  Value=double(1)  OutDataTypeStr=boolean  SampleTime=1e-08
  Unit Delay Enabled Synchronous2_lowered_ctrl_const : Constant  OutDataTypeStr=boolean  SampleTime=1e-08
  Unit Delay Enabled Synchronous2_lowered_ctrl_delay : Delay  DelayLength=double(1)  InitialCondition=0  SampleTime=1e-08
  Unit Delay Enabled Synchronous2_lowered_switch : Switch  Criteria=u2 ~= 0  Threshold=double(0)  OutDataTypeStr=boolean  SampleTime=1e-08  SaturateOnIntegerOverflow=off  InputSameDT=off
  Unit Delay Enabled Synchronous3_lowered : Delay  DelayLength=double(1)  InitialCondition=0  SampleTime=1e-08
  Unit Delay Enabled Synchronous3_lowered_Initial_Val : Constant  Value=double(1)  OutDataTypeStr=boolean  SampleTime=1e-08
  Unit Delay Enabled Synchronous3_lowered_ctrl_const : Constant  OutDataTypeStr=boolean  SampleTime=1e-08
  Unit Delay Enabled Synchronous3_lowered_ctrl_delay : Delay  DelayLength=double(1)  InitialCondition=0  SampleTime=1e-08
  Unit Delay Enabled Synchronous3_lowered_switch : Switch  Criteria=u2 ~= 0  Threshold=double(0)  OutDataTypeStr=boolean  SampleTime=1e-08  SaturateOnIntegerOverflow=off  InputSameDT=off
  Unit Delay Enabled Synchronous_lowered : Delay  DelayLength=double(1)  InitialCondition=0  SampleTime=1e-08
  Unit Delay Enabled Synchronous_lowered_Initial_Val : Constant  Value=double(1)  OutDataTypeStr=boolean  SampleTime=1e-08
  Unit Delay Enabled Synchronous_lowered_ctrl_const : Constant  OutDataTypeStr=boolean  SampleTime=1e-08
  Unit Delay Enabled Synchronous_lowered_ctrl_delay : Delay  DelayLength=double(1)  InitialCondition=0  SampleTime=1e-08
  Unit Delay Enabled Synchronous_lowered_switch : Switch  Criteria=u2 ~= 0  Threshold=double(0)  OutDataTypeStr=boolean  SampleTime=1e-08  SaturateOnIntegerOverflow=off  InputSameDT=off
  bus_selector : BusSelector  OutputSignals=start,end,valid
  enb_in{,1..18} (19 alike) : Switch  Criteria=u2 ~= 0  Threshold=double(0)  OutDataTypeStr=boolean  SampleTime=1e-08  SaturateOnIntegerOverflow=off  InputSameDT=off
  reset_in{,1..18} (19 alike) : Switch  Criteria=u2 ~= 0  Threshold=double(0)  OutDataTypeStr=boolean  SampleTime=1e-08  SaturateOnIntegerOverflow=off  InputSameDT=off
  t : Demux
  data_out : Outport  SampleTime=1e-08
  ctrl_out : Outport  Port=2  SampleTime=1e-08
  wires:
  data_in/1 -> Delay1/1
  ctrl_in/1 -> bus_selector/1
  SI/1 -> t/1
  bus_selector/1 -> Goto3/1, Delay3/1  "<start>"
  bus_selector/2 -> Delay4/1  "<end>"
  bus_selector/3 -> Goto2/1, Delay5/1  "<valid>"
  Delay1/1 -> Logical Operator/1
  Delay3/1 -> Sample Control Bus Creator/1
  Delay4/1 -> Sample Control Bus Creator/2
  Delay5/1 -> Sample Control Bus Creator/3
  Logical Operator/1 -> data_out/1
  Logical Operator1/1 -> Logical Operator/2, Switch/3
  Sample Control Bus Creator/1 -> ctrl_out/1
  Goto2/1 -> From8/1, From6/1, From44/1, From42/1, From40/1, From4/1, From38/1, From36/1, From34/1, From32/1, From30/1, From28/1, From26/1, From24/1, From22/1, From20/1, From2/1, From18/1, From16/1, From14/1, From12/1, From10/1, From/1
  Goto3/1 -> From9/1, From7/1, From5/1, From45/1, From43/1, From41/1, From39/1, From37/1, From35/1, From33/1, From31/1, From3/1, From29/1, From27/1, From25/1, From23/1, From21/1, From19/1, From17/1, From15/1, From13/1, From11/1, From1/1
  C10_lowered_ctrl_const/1 -> C10_lowered_ctrl_delay/1
  C11_lowered_ctrl_const/1 -> C11_lowered_ctrl_delay/1
  C12_lowered_ctrl_const/1 -> C12_lowered_ctrl_delay/1
  C13_lowered_ctrl_const/1 -> C13_lowered_ctrl_delay/1
  C14_lowered_ctrl_const/1 -> C14_lowered_ctrl_delay/1
  C15_lowered_ctrl_const/1 -> C15_lowered_ctrl_delay/1
  C16_lowered_ctrl_const/1 -> C16_lowered_ctrl_delay/1
  C17_lowered_ctrl_const/1 -> C17_lowered_ctrl_delay/1
  C18_lowered_ctrl_const/1 -> C18_lowered_ctrl_delay/1
  C19_lowered_ctrl_const/1 -> C19_lowered_ctrl_delay/1
  C20_lowered_ctrl_const/1 -> C20_lowered_ctrl_delay/1
  C21_lowered_ctrl_const/1 -> C21_lowered_ctrl_delay/1
  C22_lowered_ctrl_const/1 -> C22_lowered_ctrl_delay/1
  C23_lowered_ctrl_const/1 -> C23_lowered_ctrl_delay/1
  C5_lowered_ctrl_const/1 -> C5_lowered_ctrl_delay/1
  C6_lowered_ctrl_const/1 -> C6_lowered_ctrl_delay/1
  C7_lowered_ctrl_const/1 -> C7_lowered_ctrl_delay/1
  C8_lowered_ctrl_const/1 -> C8_lowered_ctrl_delay/1
  C9_lowered_ctrl_const/1 -> C9_lowered_ctrl_delay/1
  Unit Delay Enabled Synchronous_lowered_ctrl_const/1 -> Unit Delay Enabled Synchronous_lowered_ctrl_delay/1
  Unit Delay Enabled Synchronous1_lowered_ctrl_const/1 -> Unit Delay Enabled Synchronous1_lowered_ctrl_delay/1
  Unit Delay Enabled Synchronous2_lowered_ctrl_const/1 -> Unit Delay Enabled Synchronous2_lowered_ctrl_delay/1
  Unit Delay Enabled Synchronous3_lowered_ctrl_const/1 -> Unit Delay Enabled Synchronous3_lowered_ctrl_delay/1
  Unit Delay Enabled Synchronous3_lowered/1 -> Unit Delay Enabled Synchronous3_lowered_switch/1
  Unit Delay Enabled Synchronous_lowered/1 -> Unit Delay Enabled Synchronous_lowered_switch/1
  Unit Delay Enabled Synchronous1_lowered/1 -> Unit Delay Enabled Synchronous1_lowered_switch/1
  Unit Delay Enabled Synchronous2_lowered/1 -> Unit Delay Enabled Synchronous2_lowered_switch/1
  C5_lowered/1 -> C5_lowered_switch/1
  C6_lowered/1 -> C6_lowered_switch/1
  C7_lowered/1 -> C7_lowered_switch/1
  C8_lowered/1 -> C8_lowered_switch/1
  C9_lowered/1 -> C9_lowered_switch/1
  C10_lowered/1 -> C10_lowered_switch/1
  C11_lowered/1 -> C11_lowered_switch/1
  C12_lowered/1 -> C12_lowered_switch/1
  C13_lowered/1 -> C13_lowered_switch/1
  C14_lowered/1 -> C14_lowered_switch/1
  C15_lowered/1 -> C15_lowered_switch/1
  C16_lowered/1 -> C16_lowered_switch/1
  C17_lowered/1 -> C17_lowered_switch/1
  C18_lowered/1 -> C18_lowered_switch/1
  C19_lowered/1 -> C19_lowered_switch/1
  C20_lowered/1 -> C20_lowered_switch/1
  C21_lowered/1 -> C21_lowered_switch/1
  C22_lowered/1 -> C22_lowered_switch/1
  C23_lowered/1 -> C23_lowered_switch/1
  t/1 -> Switch/1
  From1/1 -> Switch/2
  From/1 -> Delay_Switch/2
  Unit Delay Enabled Synchronous3_lowered_ctrl_delay/1 -> Unit Delay Enabled Synchronous3_lowered_switch/2
  Unit Delay Enabled Synchronous3_lowered_Initial_Val/1 -> Unit Delay Enabled Synchronous3_lowered_switch/3
  t/2 -> Switch1/1
  From3/1 -> Switch1/2
  From2/1 -> Delay_Switch1/2
  Unit Delay Enabled Synchronous_lowered_ctrl_delay/1 -> Unit Delay Enabled Synchronous_lowered_switch/2
  Unit Delay Enabled Synchronous_lowered_Initial_Val/1 -> Unit Delay Enabled Synchronous_lowered_switch/3
  t/3 -> Switch2/1
  From7/1 -> Switch2/2
  From4/1 -> Delay_Switch2/2
  Unit Delay Enabled Synchronous1_lowered_ctrl_delay/1 -> Unit Delay Enabled Synchronous1_lowered_switch/2
  Unit Delay Enabled Synchronous1_lowered_Initial_Val/1 -> Unit Delay Enabled Synchronous1_lowered_switch/3
  t/4 -> Switch3/1
  From5/1 -> Switch3/2
  From6/1 -> Delay_Switch3/2
  Unit Delay Enabled Synchronous2_lowered_ctrl_delay/1 -> Unit Delay Enabled Synchronous2_lowered_switch/2
  Unit Delay Enabled Synchronous2_lowered_Initial_Val/1 -> Unit Delay Enabled Synchronous2_lowered_switch/3
  From8/1 -> enb_in/2
  Initial_Val14/1 -> reset_in/1
  From9/1 -> reset_in/2
  C5_lowered_ctrl_delay/1 -> C5_lowered_switch/2
  C5_lowered_Initial_Val/1 -> C5_lowered_switch/3
  From10/1 -> enb_in1/2
  Initial_Val15/1 -> reset_in1/1
  From11/1 -> reset_in1/2
  C6_lowered_ctrl_delay/1 -> C6_lowered_switch/2
  C6_lowered_Initial_Val/1 -> C6_lowered_switch/3
  From12/1 -> enb_in2/2
  Initial_Val16/1 -> reset_in2/1
  From13/1 -> reset_in2/2
  C7_lowered_ctrl_delay/1 -> C7_lowered_switch/2
  C7_lowered_Initial_Val/1 -> C7_lowered_switch/3
  From14/1 -> enb_in3/2
  Initial_Val17/1 -> reset_in3/1
  From15/1 -> reset_in3/2
  C8_lowered_ctrl_delay/1 -> C8_lowered_switch/2
  C8_lowered_Initial_Val/1 -> C8_lowered_switch/3
  From16/1 -> enb_in4/2
  Initial_Val18/1 -> reset_in4/1
  From17/1 -> reset_in4/2
  C9_lowered_ctrl_delay/1 -> C9_lowered_switch/2
  C9_lowered_Initial_Val/1 -> C9_lowered_switch/3
  From24/1 -> enb_in5/2
  Initial_Val/1 -> reset_in5/1
  From25/1 -> reset_in5/2
  C10_lowered_ctrl_delay/1 -> C10_lowered_switch/2
  C10_lowered_Initial_Val/1 -> C10_lowered_switch/3
  From26/1 -> enb_in6/2
  Initial_Val1/1 -> reset_in6/1
  From27/1 -> reset_in6/2
  C11_lowered_ctrl_delay/1 -> C11_lowered_switch/2
  C11_lowered_Initial_Val/1 -> C11_lowered_switch/3
  From28/1 -> enb_in7/2
  Initial_Val2/1 -> reset_in7/1
  From29/1 -> reset_in7/2
  C12_lowered_ctrl_delay/1 -> C12_lowered_switch/2
  C12_lowered_Initial_Val/1 -> C12_lowered_switch/3
  From30/1 -> enb_in8/2
  Initial_Val3/1 -> reset_in8/1
  From31/1 -> reset_in8/2
  C13_lowered_ctrl_delay/1 -> C13_lowered_switch/2
  C13_lowered_Initial_Val/1 -> C13_lowered_switch/3
  From18/1 -> enb_in9/2
  Initial_Val4/1 -> reset_in9/1
  From19/1 -> reset_in9/2
  C14_lowered_ctrl_delay/1 -> C14_lowered_switch/2
  C14_lowered_Initial_Val/1 -> C14_lowered_switch/3
  From20/1 -> enb_in10/2
  Initial_Val5/1 -> reset_in10/1
  From21/1 -> reset_in10/2
  C15_lowered_ctrl_delay/1 -> C15_lowered_switch/2
  C15_lowered_Initial_Val/1 -> C15_lowered_switch/3
  From22/1 -> enb_in11/2
  Initial_Val6/1 -> reset_in11/1
  From23/1 -> reset_in11/2
  C16_lowered_ctrl_delay/1 -> C16_lowered_switch/2
  C16_lowered_Initial_Val/1 -> C16_lowered_switch/3
  From38/1 -> enb_in12/2
  Initial_Val7/1 -> reset_in12/1
  From39/1 -> reset_in12/2
  C17_lowered_ctrl_delay/1 -> C17_lowered_switch/2
  C17_lowered_Initial_Val/1 -> C17_lowered_switch/3
  From40/1 -> enb_in13/2
  Initial_Val8/1 -> reset_in13/1
  From41/1 -> reset_in13/2
  C18_lowered_ctrl_delay/1 -> C18_lowered_switch/2
  C18_lowered_Initial_Val/1 -> C18_lowered_switch/3
  From42/1 -> enb_in14/2
  Initial_Val9/1 -> reset_in14/1
  From43/1 -> reset_in14/2
  C19_lowered_ctrl_delay/1 -> C19_lowered_switch/2
  C19_lowered_Initial_Val/1 -> C19_lowered_switch/3
  From44/1 -> enb_in15/2
  Initial_Val10/1 -> reset_in15/1
  From45/1 -> reset_in15/2
  C20_lowered_ctrl_delay/1 -> C20_lowered_switch/2
  C20_lowered_Initial_Val/1 -> C20_lowered_switch/3
  From32/1 -> enb_in16/2
  Initial_Val11/1 -> reset_in16/1
  From33/1 -> reset_in16/2
  C21_lowered_ctrl_delay/1 -> C21_lowered_switch/2
  C21_lowered_Initial_Val/1 -> C21_lowered_switch/3
  From34/1 -> enb_in17/2
  Initial_Val12/1 -> reset_in17/1
  From35/1 -> reset_in17/2
  C22_lowered_ctrl_delay/1 -> C22_lowered_switch/2
  C22_lowered_Initial_Val/1 -> C22_lowered_switch/3
  From36/1 -> enb_in18/2
  Initial_Val13/1 -> reset_in18/1
  From37/1 -> reset_in18/2
  C23_lowered_ctrl_delay/1 -> C23_lowered_switch/2
  C23_lowered_Initial_Val/1 -> C23_lowered_switch/3
  Delay_Switch/1 -> Unit Delay Enabled Synchronous3_lowered/1
  Delay_Switch1/1 -> Unit Delay Enabled Synchronous_lowered/1
  Delay_Switch2/1 -> Unit Delay Enabled Synchronous1_lowered/1
  Delay_Switch3/1 -> Unit Delay Enabled Synchronous2_lowered/1
  reset_in/1 -> C5_lowered/1
  reset_in1/1 -> C6_lowered/1
  reset_in2/1 -> C7_lowered/1
  reset_in3/1 -> C8_lowered/1
  reset_in4/1 -> C9_lowered/1
  reset_in5/1 -> C10_lowered/1
  reset_in6/1 -> C11_lowered/1
  reset_in7/1 -> C12_lowered/1
  reset_in8/1 -> C13_lowered/1
  reset_in9/1 -> C14_lowered/1
  reset_in10/1 -> C15_lowered/1
  reset_in11/1 -> C16_lowered/1
  reset_in12/1 -> C17_lowered/1
  reset_in13/1 -> C18_lowered/1
  reset_in14/1 -> C19_lowered/1
  reset_in15/1 -> C20_lowered/1
  reset_in16/1 -> C21_lowered/1
  reset_in17/1 -> C22_lowered/1
  reset_in18/1 -> C23_lowered/1
  Switch/1 -> Delay_Switch/1
  Unit Delay Enabled Synchronous3_lowered_switch/1 -> Switch1/3, Delay_Switch/3
  Switch1/1 -> Delay_Switch1/1
  Unit Delay Enabled Synchronous_lowered_switch/1 -> Switch2/3, Delay_Switch1/3
  Switch2/1 -> Delay_Switch2/1
  Unit Delay Enabled Synchronous1_lowered_switch/1 -> Switch3/3, Delay_Switch2/3
  Switch3/1 -> Delay_Switch3/1
  Unit Delay Enabled Synchronous2_lowered_switch/1 -> Delay_Switch3/3, enb_in/1
  enb_in/1 -> reset_in/3
  C5_lowered_switch/1 -> enb_in1/1, enb_in/3
  enb_in1/1 -> reset_in1/3
  C6_lowered_switch/1 -> enb_in2/1, enb_in1/3
  enb_in2/1 -> reset_in2/3
  C7_lowered_switch/1 -> enb_in3/1, enb_in2/3
  enb_in3/1 -> reset_in3/3
  C8_lowered_switch/1 -> enb_in4/1, enb_in3/3
  enb_in4/1 -> reset_in4/3
  C9_lowered_switch/1 -> enb_in4/3, enb_in5/1
  enb_in5/1 -> reset_in5/3
  C10_lowered_switch/1 -> enb_in6/1, enb_in5/3
  enb_in6/1 -> reset_in6/3
  C11_lowered_switch/1 -> enb_in7/1, enb_in6/3
  enb_in7/1 -> reset_in7/3
  C12_lowered_switch/1 -> enb_in8/1, enb_in7/3
  enb_in8/1 -> reset_in8/3
  C13_lowered_switch/1 -> enb_in9/1, enb_in8/3
  enb_in9/1 -> reset_in9/3
  C14_lowered_switch/1 -> enb_in10/1, enb_in9/3
  enb_in10/1 -> reset_in10/3
  C15_lowered_switch/1 -> enb_in11/1, enb_in10/3
  enb_in11/1 -> reset_in11/3
  C16_lowered_switch/1 -> enb_in12/1, enb_in11/3
  enb_in12/1 -> reset_in12/3
  C17_lowered_switch/1 -> enb_in13/1, enb_in12/3
  enb_in13/1 -> reset_in13/3
  C18_lowered_switch/1 -> Logical Operator1/2, enb_in14/1, enb_in13/3
  enb_in14/1 -> reset_in14/3
  C19_lowered_switch/1 -> enb_in15/1, enb_in14/3
  enb_in15/1 -> reset_in15/3
  C20_lowered_switch/1 -> enb_in16/1, enb_in15/3
  enb_in16/1 -> reset_in16/3
  C21_lowered_switch/1 -> enb_in17/1, enb_in16/3
  enb_in17/1 -> reset_in17/3
  C22_lowered_switch/1 -> enb_in18/1, enb_in17/3
  enb_in18/1 -> reset_in18/3
  C23_lowered_switch/1 -> Logical Operator1/1, enb_in18/3

== system my_gm_HDLPayloadFull/payload_full/payload_rep ==
  data_in : Inport  OutDataTypeStr=boolean  SampleTime=1e-08
  ctrl_in : Inport  Port=2  SampleTime=1e-08
  data_out : Outport  SampleTime=1e-08
  ctrl_out : Outport  Port=2  SampleTime=1e-08
  wires:
  data_in/1 -> data_out/1
  ctrl_in/1 -> ctrl_out/1
